simulink model "model"  (R2023b)
settings: Solver=VariableStepAuto  StartTime=0.0  StopTime=10.0  RelTol=1e-3
settings Model: Creator=fabio  LastModifiedBy=fabio

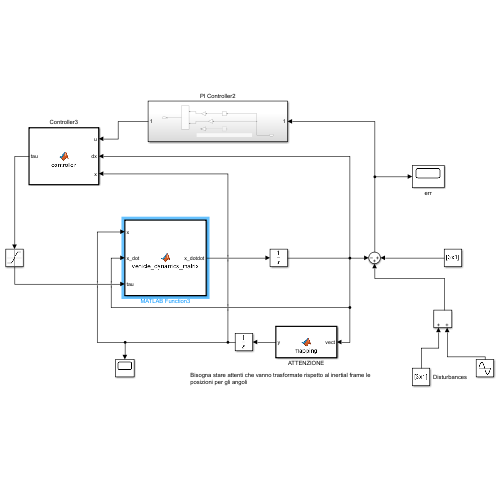
[thumbnail: Simulink's stored preview of the top-level diagram]
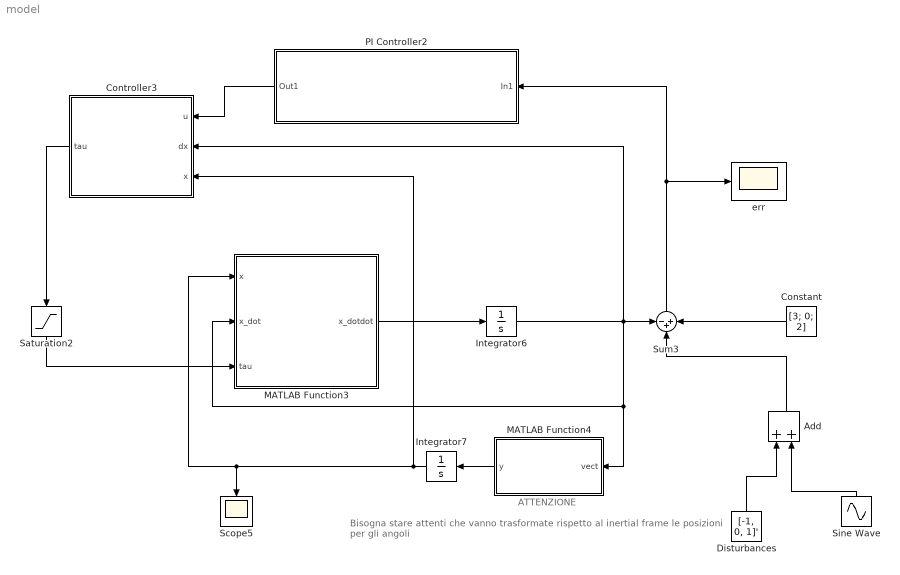
== system model ==
  note: Bisogna stare attenti che vanno trasformate rispetto al inertial frame le posizioni per gli angoli
  note: ATTENZIONE
  Add : Sum
  Constant : Constant  Value=[3; 0; 2]
  Controller3 : MATLAB Function  TreatAsAtomicUnit=on
  Disturbances : Constant  Value=[-1, 0, 1]'
  Integrator6 : Integrator
  Integrator7 : Integrator
  MATLAB Function3 : MATLAB Function  TreatAsAtomicUnit=on
  MATLAB Function4 : MATLAB Function  TreatAsAtomicUnit=on
  PI Controller2 : Subsystem
  Saturation2 : Saturate  UpperLimit=20000  LowerLimit=-20000
  Scope5 : Scope
  Sine Wave : Sin  Amplitude=0.1  Frequency=0.05  SampleTime=0
  Sum3 : Sum  Inputs=-++
  err : Scope
  wires:
  Sum3/1 -> PI Controller2/1(In1), err/1
  Saturation2/1 -> MATLAB Function3/3(tau)
  PI Controller2/1(Out1) -> Controller3/1(u)
  Integrator6/1 -> MATLAB Function4/1(vect), MATLAB Function3/2(x_dot), Controller3/2(dx), Sum3/1
  MATLAB Function3/1(x_dotdot) -> Integrator6/1
  Integrator7/1 -> Controller3/3(x), MATLAB Function3/1(x), Scope5/1
  Controller3/1(tau) -> Saturation2/1
  MATLAB Function4/1(y) -> Integrator7/1
  Disturbances/1 -> Add/1
  Add/1 -> Sum3/2
  Sine Wave/1 -> Add/2
  Constant/1 -> Sum3/3

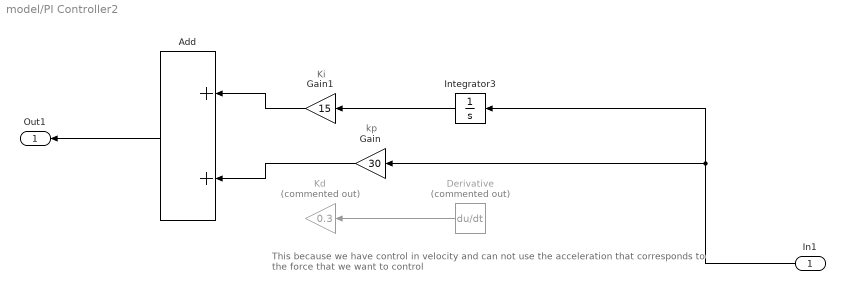
== system model/PI Controller2 ==
  note: This because we have control in velocity and can not use the acceleration that corresponds to the force that we want to control
  note: Ki
  note: kp
  In1 : Inport
  Add : Sum
  Derivative : Derivative  Commented=on
  Gain : Gain  Gain=30
  Gain1 : Gain  Gain=15
  Integrator3 : Integrator
  Kd : Gain  Commented=on  Gain=0.3
  Out1 : Outport
  wires:
  Derivative/1 -> Kd/1
  Gain/1 -> Add/2
  Integrator3/1 -> Gain1/1
  In1/1 -> Integrator3/1, Gain/1
  Add/1 -> Out1/1
  Gain1/1 -> Add/1

== matlab function model/Controller3 ==
  data: u input; dx input; tau output; x input
function tau = controller(u, dx, x)
    % updated to medusa model
    m = 30;
    I = 4.14;
    K = 1;
    g = 9.81;
    B = 0; % Buoyancy

    % Added mass
    tau_a = [-25; -2.325; -8.690; 0]; % kl_dot

    % Restoring forces
    tau_r = [-0.2; -55.117; -4.14; 0]; % kl

    % Hydrodynamic forces
    tau_d = [-19.5; -147.9; -6.23; 0]; % kl_modl

    % Virtual mass
    mv = [m; m; I; m] - tau_a;

    % Dissatipative forces
    dv = -tau_r - tau_d .* abs(dx);

    % Accelerations
    %% 3 DOF MODEL
    tau = zeros(4,1);
    tau(1) = mv(1)*K*u(1) - mv(2)*dx(2)*dx(3) + dv(1)*dx(1);
    % tau(2) = mv(2)*K*u(2) + mv(2)*dx(1)*dx(3) + dv(2)*dx(2);
    tau(3) = mv(3)*K*u(3) - (mv(1) - mv(2))*dx(1)*dx(2) + dv(3)*dx(3);
    % Considering also depth (heavy)
    % tau(4) =  mv(4)*K*u(4) + dv(3)*dx(3) - (m*g - B);

end

== matlab function model/MATLAB Function3 ==
  data: x input; x_dot input; tau input; x_dotdot output
function x_dotdot = vehicle_dynamics_matrix(x, x_dot, tau)
    % updated to medusa model
    m = 30;
    I = 4.14;
    g = 9.81;
    B = 0; % Buoyancy

    % Added mass
    tau_a = [-25; -2.325; -8.690; 0]; % kl_dot

    % Restoring forces
    tau_r = [-0.2; -55.117; -4.14; 0]; % kl

    % Hydrodynamic forces
    tau_d = [-19.5; -147.9; -6.23; 0]; % kl_modl

    % Virtual mass
    mv = [m; m; I; m] - tau_a;

    % Dissatipative forces
    dv = -tau_r - tau_d .* abs(x_dot);

    % Accelerations
    %% 3 DOF MODEL
    x_dotdot = zeros(4,1);
    tau(2) = 0; % to respect always the condition of under actuation
    x_dotdot(1) = (tau(1) + mv(2)*x_dot(2)*x_dot(3) - dv(1)*x_dot(1)) / mv(1); 
    x_dotdot(2) = (tau(2) - mv(1)*x_dot(1)*x_dot(3) - dv(2)*x_dot(2)) / mv(2);
    x_dotdot(3) = (tau(3) + (mv(1) - mv(2))*x_dot(1)*x_dot(2) - dv(3)*x_dot(3)) / mv(3);
    % Considering also depth (heavy)
    % x_dotdot(4) = (tau(4) - dv(4)*x_dot(4) + (m*g - B)) / mv(4);

== matlab function model/MATLAB Function4 ==
  data: y output; vect input
function y = mapping(vect)
    % Transformation from body farme to inertial frame of velocities
    % Migliora mettendo la vera jacobiana 
    y = zeros(3,1);
    y(1) = vect(1) * cos(vect(3)) - vect(2) * sin(vect(3));
    y(2) = vect(1) * sin(vect(3)) + vect(2) * cos(vect(3));
    y(3) = vect(3);
    % aggiungi depth
    % y(4) = vect(4);
end
